simulink model "wahadlo_online"  (Simulink 7.3)
settings: Solver=ode45  StartTime=0.0  StopTime=inf  MaxStep=0.01  RelTol=1e-3
settings Model: Creator=mklepacki  LastModifiedBy=psoltysiak

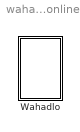
== system wahadlo_online ==
  Wahadlo : Subsystem  mask{m=10, l=3, g=9.81, fi0=179, k=0, to=0.1}
      mask prompts: m "masa"; l "dlugosc"; g "przyspieszenie"; fi0 "kat"; k "wsp tlum"; to "czas odswierzania"

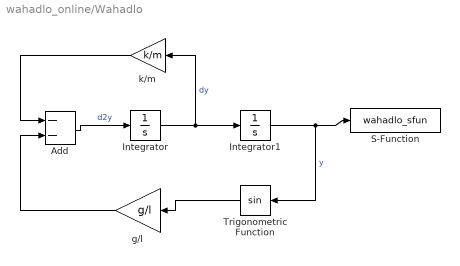
== system wahadlo_online/Wahadlo ==
  Add : Sum  Inputs=--  OutDataType=fixdt(1, 16)  OutScaling=2^-10
  Integrator : Integrator
  Integrator1 : Integrator  InitialCondition=fi0*pi/180
  S-Function : S-Function  FunctionName=wahadlo_sfun  Parameters=l,m,fi0,to  EnableBusSupport=off
  Trigonometric Function : Trigonometry
  g/l : Gain  Gain=g/l  ParameterDataType=fixdt(1, 16)  ParameterScaling=2^0  OutDataType=fixdt(1, 16)  OutScaling=2^0
  k/m : Gain  Gain=k/m  ParameterDataType=fixdt(1, 16)  ParameterScaling=2^0  OutDataType=fixdt(1, 16)  OutScaling=2^0
  wires:
  Add/1 -> Integrator/1  "d2y"
  Integrator/1 -> Integrator1/1, k/m/1  "dy"
  Integrator1/1 -> Trigonometric Function/1, S-Function/1  "y"
  Trigonometric Function/1 -> g/l/1
  k/m/1 -> Add/1
  g/l/1 -> Add/2
